simulink model "TailSitter_waypoints"  (R2018b)
settings: Solver=VariableStepAuto  StartTime=0.0  StopTime=500  RelTol=1e-3
values from neighbouring files (symbols this model uses):
  p =     [ds.mat]    (also in vxs.mat)
undefined symbols (not defined in the file or in its folder): quatnormalize
libraries: aerolibutil x18, simulink x8, sharedtransform x4, vrlib x3, sharedutil x3, simulink_extras x2, peGeneralControl x1, aerolibanim x1, aerolibanimutils x1
(part 2 of 2)

== matlab function TailSitter_waypoints/linegenerator ==
  settings: updateMethod=DISCRETE
  data: max2l input; d2lcoeff input; v_wf input; r input; altError output; p parameter; rspeed output; refvec output; wpN output; dist2wp output; thetastar output; theta output; vec2line output
function [altError, rspeed, refvec, wpN, dist2wp, thetastar, theta, vec2line] = LineGenerator(max2l, d2lcoeff, v_wf,r,p)

% Keep track of which waypoint we are going to
persistent waypointno;
persistent wp;
persistent wp_prev;
if isempty(waypointno)
    waypointno = 2;
    wp = p.waypoints(waypointno,:)';
    wp_prev = p.waypoints(waypointno-1,:)';
end

%initialize variables
dist2line2d = 0;
altError = 0;
thetaerr = 0;
rspeed = 0;
vec2line = [0,0,0]';

% if current waypoint is the start wp/home wp jump immediately to next.
dist2wp = sqrt( sum( (wp(1:3)-r).^2 ) );
if dist2wp <= p.wpradius
    if waypointno < p.numwp
        waypointno = waypointno+1;
    else
        waypointno = 2; % we always skip home wp at origin
    end
    wp_prev = wp;
    wp = p.waypoints(waypointno,:)';
end
rspeed = wp(4);

% find vector between last waypoint and current target
linevec = (wp(1:3)-wp_prev(1:3))./sqrt( sum((wp(1:3)-wp_prev(1:3)).^2) );

% Figure out if goal is ahead of us or if we passed it/missed it.
%if dot(v_wf(1:3), wp(1:3)-r(1:3)) < 0
%    linevec(1:2) = - linevec(1:2);
%end
% THe above doesn't work.

% find angle in x-y plane of vector
thetastar = atan2(linevec(2), linevec(1));
% find our current heading
theta = atan2(v_wf(2),v_wf(1));
% Error in direction along line / be paralell with line
thetaerr = thetastar - theta;


% Find the vector that describes the vector to the closest point on the
% line
a = wp_prev(1:3);
n = linevec;
vec2line = a-r - dot(a-r,n)*n;
altError = vec2line(3);
dist2line2d = sqrt( sum( vec2line(1:2).^2 ));
wpN = waypointno;


% Mix the vectors for reference according to how far away from line we are
%cr = cross(linevec,vec2line);
%refvec = linevec;
if abs(d2lcoeff*dist2line2d) < max2l
    refvec = linevec + d2lcoeff*dist2line2d*vec2line;
else
    refvec = linevec + max2l*vec2line;
end
refvec = refvec/sqrt(sum(refvec.^2));

== matlab function TailSitter_waypoints/AdHoc1 ==
  data: u_omegaL output; u_omegaR output; u_deltaL output; u_deltaR output; tx input; ty input; tz input; u_jointT input
function [u_omegaL,u_omegaR, u_deltaL,u_deltaR]  = AdHocTorques(tx, ty, tz, u_jointT)


u_deltaL = 0;
u_deltaR = 0;
u_omegaL = 0;
u_omegaR = 0;



u_deltaA = -tx;
u_jointA = -ty;
u_deltaT = -tz;

u_deltaL = u_jointA - u_deltaA/2;
u_deltaR = u_jointA + u_deltaA/2;
u_omegaL = u_jointT + u_deltaT/2;
u_omegaR = u_jointT - u_deltaT/2;


end

== matlab function TailSitter_waypoints/MATLAB Function3 ==
  data: yaw output; vr_wf input; pitch output; yawr output; v_wf input; pitchPID input
function [yaw, pitch, yawr] = fcn(vr_wf, v_wf, pitchPID)

yawe = 0;
pitch = 0;
yawr = 0;

% Angle toward horizon given by:
horzspeedr = sqrt(sum(vr_wf(1:2).^2));
pitch = (horzspeedr +6.013)/15.38;
% correct for coordsys of pitch
pitch = (pi/2-pitch);

% correct pitch using measurments, use external pid
pitch = pitch + pitchPID;

% reference heading
yawr = atan2(vr_wf(2),vr_wf(1));
%current heading
yaw = atan2(v_wf(2),v_wf(1));

% use error in direction to roll slightly, use external PID
%roll = 0.1*yawe;

== matlab function TailSitter_waypoints/pitchError ==
  data: vr_wf input; vherror output; v_wf input; horzspeedr output; horzspeed output
function [vherror,horzspeedr, horzspeed]  = pitchError(vr_wf, v_wf)


% Angle toward horizon given by:
horzspeedr = sqrt(sum(vr_wf(1:2).^2));
horzspeed  = sqrt(sum( v_wf(1:2).^2));

vherror = horzspeedr-horzspeed;

== matlab function TailSitter_waypoints/linegenerator_old ==
  settings: updateMethod=DISCRETE
  data: v_wf input; dist2line2d output; r input; altError output; p parameter; thetaerr output; rspeed output; linevec output; vec2line output; wpN output
function [dist2line2d,altError, thetaerr, rspeed, linevec, vec2line, wpN] = LineGenerator(v_wf,r,p)

% Keep track of which waypoint we are going to
persistent waypointno;
persistent wp;
persistent wp_prev;
if isempty(waypointno)
    waypointno = 2;
    wp = p.waypoints(waypointno,:)';
    wp_prev = p.waypoints(waypointno-1,:)';
end

%initialize variables
dist2line2d = 0;
altError = 0;
thetaerr = 0;
rspeed = 0;
vec2line = [0,0,0]';

% if current waypoint is the start wp/home wp jump immediately to next.
if sqrt( sum( (wp(1:3)-r).^2 ) ) <= p.wpradius
    if waypointno < p.numwp
        waypointno = waypointno+1;
    else
        waypointno = 2; % we always skip home wp at origin
    end
    wp_prev = wp;
    wp = p.waypoints(waypointno,:)';
end
rspeed = wp(4);

% find vector between last waypoint and current target
linevec = (wp(1:3)-wp_prev(1:3))./sqrt( sum((wp(1:3)-wp_prev(1:3)).^2) );

% Figure out if goal is ahead of us or if we passed it/missed it.
%if dot(v_wf(1:3), wp(1:3)-r(1:3)) < 0
%    linevec(1:2) = - linevec(1:2);
%end
% THe above doesn't work. lets start discretizing instead

% find angle in x-y plane of vector
thetastar = atan2(linevec(2), linevec(1));
% find our current heading
theta = atan2(v_wf(2),v_wf(1));
% Error in direction along line / be paralell with line
thetaerr = thetastar - theta;


% Find the vector that describes the vector to the closest point on the
% line
a = wp_prev(1:3);
n = linevec;
vec2line = a-r - dot(a-r,n)*n;
altError = vec2line(3);
dist2line2d = sqrt( sum( vec2line(1:2).^2 ));
wpN = waypointno;

== matlab function TailSitter_waypoints/MATLAB Function4 ==
  data: u input; y output
function y = fcn(u)

y = [0,0,0,0];
qa = quaternion(u', 'euler', 'ZYX', 'frame');
y = qa.compact;

== matlab function TailSitter_waypoints/MATLAB Function5 ==
  data: yawr input; yawe output; yaw input
function yawe = fcn(yawr,yaw)

% IF our angle error is more than 180 degrees we need to cross the sign
% barrier, this code should take care of that.
% Since rate limiters are in play, we might need to loo at yawr_target, but
% lets wait with that for now.

yawe = yawr-yaw;
% r:100, y:-90 => e=190 => -360+190= -170
% r:-100, y=90 => e=-190 => 360+(-190) = 170
if yawe > pi
    yawe = -2*pi+yawe;
elseif yawe < -pi
    yawe = 2*pi+yawe;
end

== matlab function TailSitter_waypoints/MATLAB Function6 ==
  data: yawr input; yawr_slow output; yawr_last input; maxrate input; p parameter
function yawr_slow  = fcn(yawr, yawr_last, maxrate, p)





% We would like to set yawr_slow to yawr, but can only approach it in steps
% of maxrate. Also take care in which direction we approach it.
yawr_slow = yawr;
e = yawr-yawr_last;
% slew rate = unit/s => (unit*sampletime)/s
maxrate = maxrate*p.Ts;

if abs(e) > maxrate
    if e > pi
        yawr_slow = yawr_last - maxrate;
    elseif e < -pi
        yawr_slow = yawr_last + maxrate;
    else
        yawr_slow = yawr_last + sign(e)*maxrate;
    end
end

while(yawr_slow > pi)
    yawr_slow = yawr_slow - 2*pi;
end
while(yawr_slow < -pi)
    yawr_slow = yawr_slow + 2*pi;
end

end
